simulink model "CruiseControlMode"  (R2022b)
settings: Solver=FixedStepDiscrete  StartTime=0.0  StopTime=10.0  FixedStep=0.01  RelTol=1e-3
undefined symbols (not defined in the file or in its folder): brake_threshold, KeyON, opMode, reqMode, ShiftDrive, tsp_max, tsp_min
libraries: simulink x46
settings Model: RequirementInfo={} %GIDa_d2754c3b_5e37_4166_8f7d_123f4ab94d38  DataDictionary=crs_controllerdic.sldd  EnableAccessToBaseWorkspace=off  Creator=The MathWorks, Inc.  LastModifiedBy=KSREERANG
settings SolverCC: AlgebraicLoopSolver=TrustRegion
settings DataIOCC: SaveOutput=off  SignalLogging=off  DSMLogging=off  SaveTime=off  ReturnWorkspaceOutputs=off
settings OptimizationCC: DefaultParameterBehavior=Inlined  PassReuseOutputArgsAs=Individual arguments  EfficientTunableParamExpr=on
settings DebuggingCC: ParameterTunabilityLossMsg=error  UnconnectedInputMsg=warning  UnconnectedOutputMsg=warning  UnconnectedLineMsg=warning  SFMachineParentedDataDiag=warning  ArithmeticOperatorsInVariantConditions=warning
settings ModelReferenceCC: EnableRefExpFcnMdlSchedulingChecks=on
settings SFSimCC: SimUseLocalCustomCode=off  CustomCodeUndefinedFunction=UseInterfaceOnly
settings RTWCC: Description=Embedded Coder  SystemTargetFile=ert.tlc  GenCodeOnly=on  TemplateMakefile=ert_default_tmf  GenerateReport=on  RTWUseLocalCustomCode=off  IncludeHyperlinkInReport=on  LaunchReport=on  GenerateTraceInfo=on  GenerateTraceReport=on  GenerateTraceReportSl=on  GenerateTraceReportSf=on  GenerateTraceReportEml=on  DLArmComputeVersion=19.05
settings CodeAppCC: ForceParamTrailComments=on  IgnoreCustomStorageClasses=off  OperatorAnnotations=on  SimulinkDataObjDesc=on  SFDataObjDesc=on  MATLABFcnDesc=on  InsertBlockDesc=on  StateflowObjectComments=on  MATLABSourceComments=on  ReqsInCode=on
settings ERTTargetCC: TargetLangStandard=C99 (ISO)  GenerateSampleERTMain=on  InlinedParameterPlacement=NonHierarchical  ERTCustomFileTemplate=example_file_process.tlc

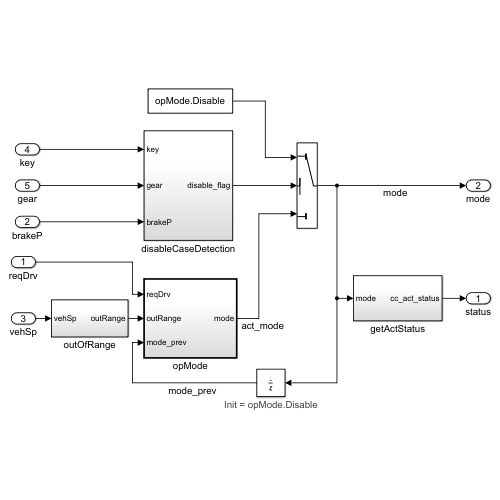
[thumbnail: Simulink's stored preview of the top-level diagram]
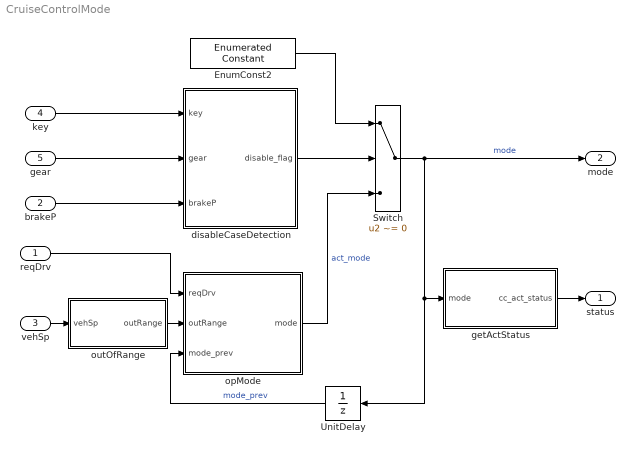
== system CruiseControlMode ==
  reqDrv : Inport  RequirementInfo={} %GIDa_e02c04ea_ec13_49e9_be49_37d1e0b933a9  OutDataTypeStr=Enum: reqMode  PortDimensions=1  SampleTime=[0.01,0]
  brakeP : Inport  RequirementInfo={} %GIDa_3b7b0db5_0c42_456e_bffc_824e0e006553  Port=2  OutDataTypeStr=double  PortDimensions=1  SampleTime=[0.01,0]
  vehSp : Inport  RequirementInfo={} %GIDa_87056838_1774_4720_931e_310af0b5e184  Port=3  OutDataTypeStr=double  PortDimensions=1  SampleTime=[0.01,0]
  key : Inport  RequirementInfo={} %GIDa_da618038_e4b4_4630_9454_d4f85815a96a  Port=4  OutDataTypeStr=uint8  PortDimensions=1  SampleTime=[0.01,0]
  gear : Inport  RequirementInfo={} %GIDa_417b91ae_b290_4c6e_bd19_c183e206983d  Port=5  OutDataTypeStr=uint8  PortDimensions=1  SampleTime=[0.01,0]
  EnumConst2 : simulink/Sources/Enumerated Constant  OutDataTypeStr=Enum: opMode  Value=opMode.Disable  SampleTime=inf
  Switch : Switch  RequirementInfo={} %GIDa_134f0e30_122b_43c5_8efc_d29582d40c21  Criteria=u2 ~= 0  SaturateOnIntegerOverflow=off  InputSameDT=off
  UnitDelay : UnitDelay  RequirementInfo={} %GIDa_6cca9198_01f1_4570_b07c_de3761ab8219  InitialCondition=opMode.Disable  SampleTime=-1  HasFrameUpgradeWarning=on
      settings: AttributesFormatString=Init = %<InitialCondition>
  disableCaseDetection : Subsystem  RequirementInfo={} %GIDa_30cfa19a_c319_430d_857b_86cf10c70b3e
  getActStatus : Subsystem  RequirementInfo={} %GIDa_922b883f_e498_4622_88f6_724ffdd11509
  opMode : Subsystem  RequirementInfo={} %GIDa_e315da79_f503_4e3a_a896_f4bec06d1909  TreatAsAtomicUnit=on
  outOfRange : Subsystem  RequirementInfo={} %GIDa_6a8018be_f3b6_456e_9531_311e94e8f57d
  status : Outport  RequirementInfo={} %GIDa_0f94b556_bb21_4013_9d6a_be506c43a1e9  OutDataTypeStr=boolean  PortDimensions=1  SampleTime=[0.01,0]  VectorParamsAs1DForOutWhenUnconnected=off
  mode : Outport  RequirementInfo={} %GIDa_cedbaee0_5a22_4a89_bb43_144b8d7ba06b  Port=2  OutDataTypeStr=Enum: opMode  PortDimensions=1  SampleTime=[0.01,0]  VectorParamsAs1DForOutWhenUnconnected=off
  wires:
  EnumConst2/1 -> Switch/1
  brakeP/1 -> disableCaseDetection/3(brakeP)
  key/1 -> disableCaseDetection/1(key)
  gear/1 -> disableCaseDetection/2(gear)
  disableCaseDetection/1(disable_flag) -> Switch/2
  reqDrv/1 -> opMode/1(reqDrv)
  UnitDelay/1 -> opMode/3(mode_prev)  "mode_prev"
  getActStatus/1(cc_act_status) -> status/1
  opMode/1(mode) -> Switch/3  "act_mode"
  Switch/1 -> UnitDelay/1, getActStatus/1(mode), mode/1  "mode"
  vehSp/1 -> outOfRange/1(vehSp)
  outOfRange/1(outRange) -> opMode/2(outRange)

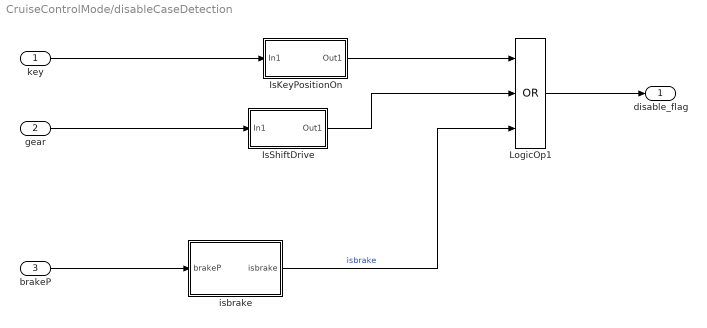
== system CruiseControlMode/disableCaseDetection ==
  key : Inport  RequirementInfo={} %GIDa_c582e8bc_b654_4724_afb0_c4fc2a3f6909
  gear : Inport  RequirementInfo={} %GIDa_4cb0485d_973c_48c3_a789_740fa1fc93bd  Port=2
  brakeP : Inport  RequirementInfo={} %GIDa_84889384_43e7_4e09_aa08_16226f740df6  Port=3
  IsKeyPositionOn : Subsystem  RequirementInfo={} %GIDa_5fa75b47_70b0_4656_b72f_350de8951d87
  IsShiftDrive : Subsystem  RequirementInfo={} %GIDa_d1da0970_5a6e_4cfb_b99c_ed1fdadca6ff
  LogicOp1 : Logic  RequirementInfo={} %GIDa_0e7638fa_faba_4642_af12_693558d1e7f2  Operator=OR  Inputs=3  AllPortsSameDT=off  OutDataTypeStr=boolean
  isbrake : Subsystem  RequirementInfo={} %GIDa_c5463be8_f4ae_4cec_a339_b8202d63dca3
  disable_flag : Outport  RequirementInfo={} %GIDa_06062790_d1b3_4bb4_a6b4_14f289277b04  VectorParamsAs1DForOutWhenUnconnected=off
  wires:
  IsShiftDrive/1(Out1) -> LogicOp1/2
  gear/1 -> IsShiftDrive/1(In1)
  IsKeyPositionOn/1(Out1) -> LogicOp1/1
  key/1 -> IsKeyPositionOn/1(In1)
  isbrake/1(isbrake) -> LogicOp1/3  "isbrake"
  brakeP/1 -> isbrake/1(brakeP)
  LogicOp1/1 -> disable_flag/1

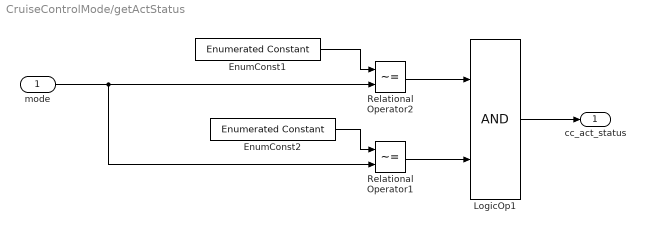
== system CruiseControlMode/getActStatus ==
  mode : Inport  RequirementInfo={} %GIDa_2327d0a8_9f89_4824_af80_f140e8b7cb64
  EnumConst1 : simulink/Sources/Enumerated Constant  RequirementInfo={} %GIDa_f8aa3c76_e1da_47ae_9bc1_37456c4f810e  OutDataTypeStr=Enum: opMode  Value=opMode.Disable  SampleTime=inf
  EnumConst2 : simulink/Sources/Enumerated Constant  RequirementInfo={} %GIDa_73c92ee3_ccad_4e01_ae3b_3441c492584d  OutDataTypeStr=Enum: opMode  Value=opMode.Enable  SampleTime=inf
  LogicOp1 : Logic  RequirementInfo={} %GIDa_d1891a75_3176_4f01_b4a6_061b63f5b5e7  AllPortsSameDT=off  OutDataTypeStr=boolean
  Relational Operator1 : RelationalOperator  RequirementInfo={} %GIDa_0ac04840_0dbf_4a47_a92d_a07906c67fea  Operator=~=  OutDataTypeStr=boolean  InputSameDT=off
  Relational Operator2 : RelationalOperator  RequirementInfo={} %GIDa_da8b8f51_89d3_4582_904d_6d29522943a4  Operator=~=  OutDataTypeStr=boolean  InputSameDT=off
  cc_act_status : Outport  RequirementInfo={} %GIDa_4f6d64e4_ebde_4261_a75c_bc573f921507  VectorParamsAs1DForOutWhenUnconnected=off
  wires:
  LogicOp1/1 -> cc_act_status/1
  EnumConst2/1 -> Relational Operator1/1
  Relational Operator1/1 -> LogicOp1/2
  mode/1 -> Relational Operator2/2, Relational Operator1/2
  EnumConst1/1 -> Relational Operator2/1
  Relational Operator2/1 -> LogicOp1/1

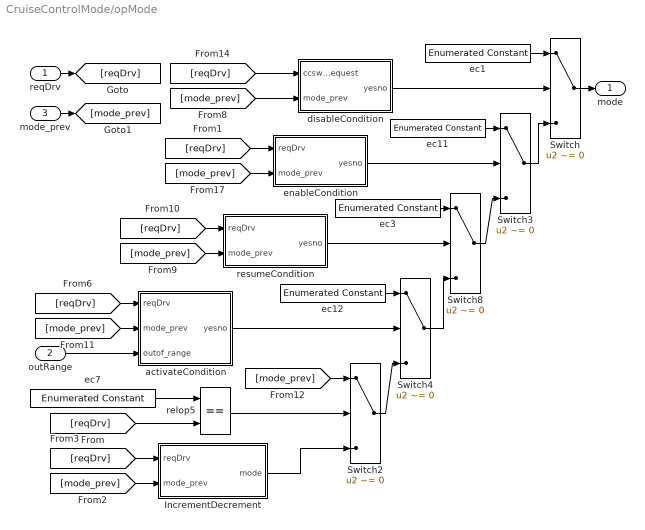
== system CruiseControlMode/opMode ==
  reqDrv : Inport  RequirementInfo={} %GIDa_d6dc1c84_5b93_4ebd_a6cb_51c4e313a83b
  outRange : Inport  RequirementInfo={} %GIDa_8f85a2d2_ead7_4273_a37e_68fc2be8b446  Port=2
  mode_prev : Inport  RequirementInfo={} %GIDa_f8adc632_9c19_43ab_ab94_9239398279c8  Port=3
  IncrementDecrement : Subsystem  RequirementInfo={} %GIDa_cf4f9597_e849_4031_bd26_eb00965c4499
  Switch : Switch  RequirementInfo={} %GIDa_f278f199_6b25_4f5b_af21_e9d29d6a7a0f  Criteria=u2 ~= 0  SaturateOnIntegerOverflow=off  InputSameDT=off
  Switch2 : Switch  RequirementInfo={} %GIDa_e275915e_0819_4e2f_a4fa_10d11a8f267d  Criteria=u2 ~= 0  SaturateOnIntegerOverflow=off  InputSameDT=off
  Switch3 : Switch  RequirementInfo={} %GIDa_e58e5032_d959_406a_99aa_4681a14fd21b  Criteria=u2 ~= 0  SaturateOnIntegerOverflow=off  InputSameDT=off
  Switch4 : Switch  RequirementInfo={} %GIDa_e86cdaa4_f011_4da8_8c69_5ad1193619c6  Criteria=u2 ~= 0  SaturateOnIntegerOverflow=off  InputSameDT=off
  Switch8 : Switch  RequirementInfo={} %GIDa_db82ae89_74d8_429e_a2c1_70767e727218  Criteria=u2 ~= 0  SaturateOnIntegerOverflow=off  InputSameDT=off
  activateCondition : Subsystem  RequirementInfo={} %GIDa_3a1937b1_e63c_4edf_b9e4_c891f61b7724
  disableCondition : Subsystem  RequirementInfo={} %GIDa_f9200ea0_df0d_4770_99ca_2bc3e49d1fe1
  ec1 : simulink/Sources/Enumerated Constant  RequirementInfo={} %GIDa_015a4b04_79f2_421f_ade4_4409e02da5c7  OutDataTypeStr=Enum: opMode  Value=opMode.Disable  SampleTime=inf
  ec11 : simulink/Sources/Enumerated Constant  RequirementInfo={} %GIDa_ec3fa4e4_42ea_4ae3_93ed_8aee2c0a39ed  OutDataTypeStr=Enum: opMode  Value=opMode.Enable  SampleTime=inf
  ec12 : simulink/Sources/Enumerated Constant  RequirementInfo={} %GIDa_fcb4c8b2_4022_407c_87a6_a915c151313b  OutDataTypeStr=Enum: opMode  Value=opMode.Activate  SampleTime=inf
  ec3 : simulink/Sources/Enumerated Constant  RequirementInfo={} %GIDa_eb9bf327_13fe_48a0_b323_af6e76e203bb  OutDataTypeStr=Enum: opMode  Value=opMode.Resume  SampleTime=inf
  ec7 : simulink/Sources/Enumerated Constant  RequirementInfo={} %GIDa_58ab4a78_7813_419b_8fc1_7974d688ddc1  OutDataTypeStr=Enum: reqMode  Value=reqMode.NoRequest  SampleTime=inf
  enableCondition : Subsystem  RequirementInfo={} %GIDa_2fd9b1f7_d568_4f68_81be_1b30c1f938c3
  relop5 : RelationalOperator  RequirementInfo={} %GIDa_b4c8cdd0_d61d_4e26_84e3_ca073b38d041  Operator===  OutDataTypeStr=boolean  InputSameDT=off
  resumeCondition : Subsystem  RequirementInfo={} %GIDa_a20f1591_47de_4d21_9f12_3ebad1f0684e
  mode : Outport  RequirementInfo={} %GIDa_b396453e_df28_4809_a65d_b57fb24c4239  VectorParamsAs1DForOutWhenUnconnected=off
  wires:
  IncrementDecrement/1(mode) -> Switch2/3
  [mode_prev] -> IncrementDecrement/2(mode_prev)
  [reqDrv] -> IncrementDecrement/1(reqDrv)
  [mode_prev] -> enableCondition/2(mode_prev)
  outRange/1 -> activateCondition/3(outof_range)
  [reqDrv] -> disableCondition/1(ccsw_request)
  ec3/1 -> Switch8/1
  [reqDrv] -> resumeCondition/1(reqDrv)
  [mode_prev] -> resumeCondition/2(mode_prev)
  resumeCondition/1(yesno) -> Switch8/2
  Switch4/1 -> Switch8/3
  Switch8/1 -> Switch3/3
  Switch2/1 -> Switch4/3
  relop5/1 -> Switch2/2
  reqDrv/1 -> [reqDrv]
  [mode_prev] -> disableCondition/2(mode_prev)
  [mode_prev] -> activateCondition/2(mode_prev)
  [reqDrv] -> activateCondition/1(reqDrv)
  activateCondition/1(yesno) -> Switch4/2
  Switch3/1 -> Switch/3
  disableCondition/1(yesno) -> Switch/2
  enableCondition/1(yesno) -> Switch3/2
  mode_prev/1 -> [mode_prev]
  [reqDrv] -> enableCondition/1(reqDrv)
  [mode_prev] -> Switch2/1
  [reqDrv] -> relop5/2
  ec12/1 -> Switch4/1
  ec11/1 -> Switch3/1
  ec7/1 -> relop5/1
  ec1/1 -> Switch/1
  Switch/1 -> mode/1

== system CruiseControlMode/outOfRange ==
  vehSp : Inport  RequirementInfo={} %GIDa_10d93d9c_c07d_4af0_b3dc_570db8225146
  Compare To Constant : simulink/Logic and Bit Operations/Compare To Constant  RequirementInfo={} %GIDa_16aaa0c8_a2f0_4c5a_ae90_6ea610de385c  relop=<  const=tsp_min  OutDataTypeStr=boolean
  Compare To Constant1 : simulink/Logic and Bit Operations/Compare To Constant  RequirementInfo={} %GIDa_bc322242_d9a7_47fb_8ec0_04de03b57b5d  relop=>  const=tsp_max  OutDataTypeStr=boolean
  LogicOp : Logic  RequirementInfo={} %GIDa_9879b928_48e1_4dc2_86e7_6ea8d95ea2bf  Operator=OR  AllPortsSameDT=off  OutDataTypeStr=boolean
  outRange : Outport  RequirementInfo={} %GIDa_05b9ac4e_46b0_439f_8ec8_ced6dca6f32b  VectorParamsAs1DForOutWhenUnconnected=off
  wires:
  vehSp/1 -> Compare To Constant1/1, Compare To Constant/1
  Compare To Constant/1 -> LogicOp/1
  Compare To Constant1/1 -> LogicOp/2
  LogicOp/1 -> outRange/1

== system CruiseControlMode/disableCaseDetection/IsKeyPositionOn ==
  In1 : Inport  RequirementInfo={} %GIDa_fbade00e_be87_4b7c_96f1_342a649bf32e
  Constant : Constant  RequirementInfo={} %GIDa_c80b2359_4f79_4558_8249_60fbc73dc217  Value=KeyON
  Relational Operator2 : RelationalOperator  RequirementInfo={} %GIDa_1085da51_22c4_4519_8a44_d44051c23fa5  Operator=~=  OutDataTypeStr=boolean  InputSameDT=off
  Out1 : Outport  RequirementInfo={} %GIDa_53421d23_320b_4638_b85c_7031813788c3  VectorParamsAs1DForOutWhenUnconnected=off
  wires:
  Constant/1 -> Relational Operator2/2
  In1/1 -> Relational Operator2/1
  Relational Operator2/1 -> Out1/1

== system CruiseControlMode/disableCaseDetection/IsShiftDrive ==
  In1 : Inport  RequirementInfo={} %GIDa_e638b041_459c_4a49_806d_2e8e8e3b1d25
  Constant1 : Constant  RequirementInfo={} %GIDa_728aeb5c_840b_4b38_9d35_2bb658e3a343  Value=ShiftDrive
  Relational Operator3 : RelationalOperator  RequirementInfo={} %GIDa_8fff1215_8b51_4cbc_a454_5baa57c7c947  Operator=~=  OutDataTypeStr=boolean  InputSameDT=off
  Out1 : Outport  RequirementInfo={} %GIDa_bd684801_c897_47ac_8c54_81cdc672ae87  VectorParamsAs1DForOutWhenUnconnected=off
  wires:
  Constant1/1 -> Relational Operator3/2
  In1/1 -> Relational Operator3/1
  Relational Operator3/1 -> Out1/1

== system CruiseControlMode/disableCaseDetection/isbrake ==
  brakeP : Inport  RequirementInfo={} %GIDa_39c608f7_59ae_4c31_a873_5a7787b80baa
  Compare To Constant : simulink/Logic and Bit Operations/Compare To Constant  RequirementInfo={} %GIDa_189ea09c_3f5c_40b7_82bc_4cba1ee5f74b  relop=>  const=brake_threshold  OutDataTypeStr=boolean
  isbrake : Outport  RequirementInfo={} %GIDa_5b8aaf44_fb4f_460a_80ba_c6eab77b7a44  VectorParamsAs1DForOutWhenUnconnected=off
  wires:
  Compare To Constant/1 -> isbrake/1
  brakeP/1 -> Compare To Constant/1

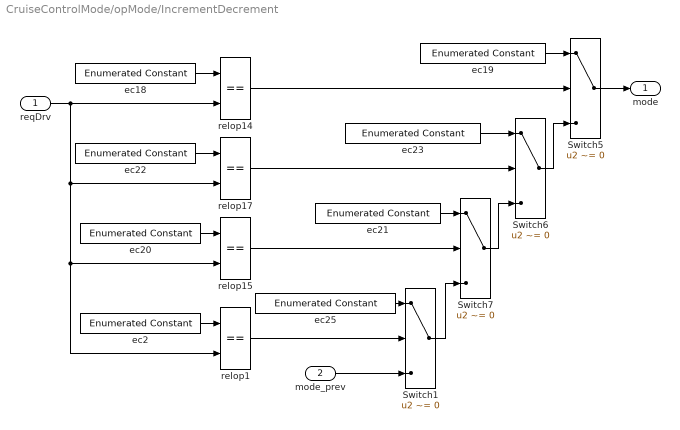
== system CruiseControlMode/opMode/IncrementDecrement ==
  reqDrv : Inport  RequirementInfo={} %GIDa_e2bc38eb_5ae3_43b9_a114_d74f24c6e37b
  mode_prev : Inport  RequirementInfo={} %GIDa_5373f4eb_c723_4fec_a619_dc0302e64efa  Port=2
  Switch1 : Switch  RequirementInfo={} %GIDa_3da03518_a025_4b01_9142_099afa888f0e  Criteria=u2 ~= 0  SaturateOnIntegerOverflow=off  InputSameDT=off
  Switch5 : Switch  RequirementInfo={} %GIDa_ad15e83e_a1a5_494f_97a5_7e76ad4b6e6a  Criteria=u2 ~= 0  SaturateOnIntegerOverflow=off  InputSameDT=off
  Switch6 : Switch  RequirementInfo={} %GIDa_d7f0e410_c4f9_4851_913e_6272620f0d58  Criteria=u2 ~= 0  SaturateOnIntegerOverflow=off  InputSameDT=off
  Switch7 : Switch  RequirementInfo={} %GIDa_76c38470_6d2c_4821_909c_522b3827856b  Criteria=u2 ~= 0  SaturateOnIntegerOverflow=off  InputSameDT=off
  ec18 : simulink/Sources/Enumerated Constant  RequirementInfo={} %GIDa_1f657265_3a4b_4f99_8045_e03baf4bd613  OutDataTypeStr=Enum: reqMode  Value=reqMode.Inc_Short  SampleTime=inf
  ec19 : simulink/Sources/Enumerated Constant  RequirementInfo={} %GIDa_da36edf3_ca28_44dd_9c44_3816caf78137  OutDataTypeStr=Enum: opMode  Value=opMode.Increment  SampleTime=inf
  ec2 : simulink/Sources/Enumerated Constant  RequirementInfo={} %GIDa_9273ddb4_1d3b_443f_98f7_4d2b24f19bc0  OutDataTypeStr=Enum: reqMode  Value=reqMode.Dec_Long  SampleTime=inf
  ec20 : simulink/Sources/Enumerated Constant  RequirementInfo={} %GIDa_795dac68_6a3a_4e07_affa_8c2c129b871d  OutDataTypeStr=Enum: reqMode  Value=reqMode.Dec_Short  SampleTime=inf
  ec21 : simulink/Sources/Enumerated Constant  RequirementInfo={} %GIDa_b5dc6f1e_17b1_4531_8089_3a1730281df9  OutDataTypeStr=Enum: opMode  Value=opMode.Decrement  SampleTime=inf
  ec22 : simulink/Sources/Enumerated Constant  RequirementInfo={} %GIDa_6acb6ee2_ef5b_4345_84a3_9181b47d18e8  OutDataTypeStr=Enum: reqMode  Value=reqMode.Inc_Long  SampleTime=inf
  ec23 : simulink/Sources/Enumerated Constant  RequirementInfo={} %GIDa_18759121_a88a_4695_aba9_877ce84448f2  OutDataTypeStr=Enum: opMode  Value=opMode.IncrementHold  SampleTime=inf
  ec25 : simulink/Sources/Enumerated Constant  RequirementInfo={} %GIDa_0fe9807b_c2cf_4c75_9774_a51ab4388cde  OutDataTypeStr=Enum: opMode  Value=opMode.DecrementHold  SampleTime=inf
  relop1 : RelationalOperator  RequirementInfo={} %GIDa_e875ba4b_a404_460a_9e1b_b0d1157735d3  Operator===  OutDataTypeStr=boolean  InputSameDT=off
  relop14 : RelationalOperator  RequirementInfo={} %GIDa_a828a7b6_80d5_4932_a549_e889a70ae76f  Operator===  OutDataTypeStr=boolean  InputSameDT=off
  relop15 : RelationalOperator  RequirementInfo={} %GIDa_a3f1fb2c_be05_49f4_b0d8_78a17c2da26b  Operator===  OutDataTypeStr=boolean  InputSameDT=off
  relop17 : RelationalOperator  RequirementInfo={} %GIDa_ea05844d_1ae3_4b99_85d9_44a8123c96a9  Operator===  OutDataTypeStr=boolean  InputSameDT=off
  mode : Outport  RequirementInfo={} %GIDa_5d5012d3_58ac_4298_b4d7_8a2f3101ae51  VectorParamsAs1DForOutWhenUnconnected=off
  wires:
  reqDrv/1 -> relop14/2, relop17/2, relop15/2, relop1/2
  Switch5/1 -> mode/1
  relop14/1 -> Switch5/2
  ec18/1 -> relop14/1
  mode_prev/1 -> Switch1/3
  relop1/1 -> Switch1/2
  ec2/1 -> relop1/1
  Switch1/1 -> Switch7/3
  ec25/1 -> Switch1/1
  Switch7/1 -> Switch6/3
  ec21/1 -> Switch7/1
  relop15/1 -> Switch7/2
  ec20/1 -> relop15/1
  Switch6/1 -> Switch5/3
  ec23/1 -> Switch6/1
  relop17/1 -> Switch6/2
  ec22/1 -> relop17/1
  ec19/1 -> Switch5/1

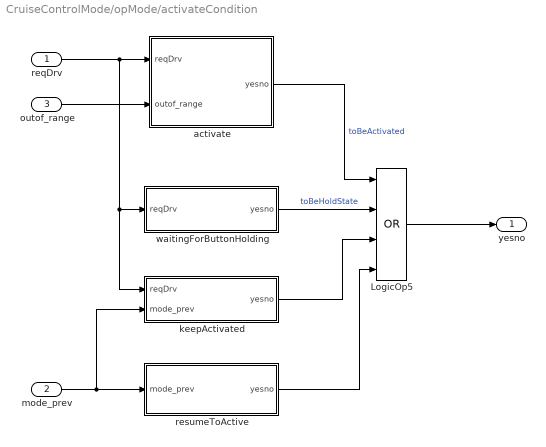
== system CruiseControlMode/opMode/activateCondition ==
  reqDrv : Inport  RequirementInfo={} %GIDa_15fdfca6_8f0c_489b_a680_659e7f1acd40
  mode_prev : Inport  RequirementInfo={} %GIDa_375ed21a_680e_4188_b39c_14c0b0419ce3  Port=2
  outof_range : Inport  RequirementInfo={} %GIDa_ccbb498a_39dc_42aa_9748_b1fab1679509  Port=3
  LogicOp5 : Logic  RequirementInfo={} %GIDa_1f1f3340_53a8_4cf3_aba1_6d6d2f2a7d3a  Operator=OR  Inputs=4  AllPortsSameDT=off  OutDataTypeStr=boolean
  activate : Subsystem  RequirementInfo={} %GIDa_ae753962_f36b_4896_8190_9ff64202b598
  keepActivated : Subsystem  RequirementInfo={} %GIDa_31cdea4a_4fb3_477d_beaa_8c8bfca90bc0
  resumeToActive : Subsystem  RequirementInfo={} %GIDa_52ef6869_8b8a_4a88_97e9_527087414cdd
  waitingForButtonHolding : Subsystem  RequirementInfo={} %GIDa_d152685c_bd82_4fc3_8902_76004ba249e5
  yesno : Outport  RequirementInfo={} %GIDa_a451725f_a3c6_4912_923c_f002f163403e  VectorParamsAs1DForOutWhenUnconnected=off
  wires:
  mode_prev/1 -> resumeToActive/1(mode_prev), keepActivated/2(mode_prev)
  resumeToActive/1(yesno) -> LogicOp5/4
  activate/1(yesno) -> LogicOp5/1  "toBeActivated"
  waitingForButtonHolding/1(yesno) -> LogicOp5/2  "toBeHoldState"
  keepActivated/1(yesno) -> LogicOp5/3
  outof_range/1 -> activate/2(outof_range)
  LogicOp5/1 -> yesno/1
  reqDrv/1 -> activate/1(reqDrv), waitingForButtonHolding/1(reqDrv), keepActivated/1(reqDrv)

== system CruiseControlMode/opMode/disableCondition ==
  ccsw_request : Inport  RequirementInfo={} %GIDa_b101258d_165d_4d04_82f5_55b581071af0
  mode_prev : Inport  RequirementInfo={} %GIDa_6cc3844b_31a9_4b0f_9f1e_2073909f59a1  Port=2
  LogicOp7 : Logic  RequirementInfo={} %GIDa_ce563152_e3e7_4710_94ca_17a1ff19942b  Operator=OR  AllPortsSameDT=off  OutDataTypeStr=boolean
  buttonsShouldBeCalledWhenActivated : Subsystem  RequirementInfo={} %GIDa_454b6547_c400_48f4_a548_bf377e739686
  turnOffCruise : Subsystem  RequirementInfo={} %GIDa_28458284_b25f_4ba6_ba6a_dfac332ba428
  yesno : Outport  RequirementInfo={} %GIDa_58737c6d_d13a_4674_9c00_2cb4f5887bd5  VectorParamsAs1DForOutWhenUnconnected=off
  wires:
  buttonsShouldBeCalledWhenActivated/1(yesno) -> LogicOp7/2
  turnOffCruise/1(yesno) -> LogicOp7/1
  mode_prev/1 -> turnOffCruise/2(mode_prev), buttonsShouldBeCalledWhenActivated/2(mode_prev)
  LogicOp7/1 -> yesno/1
  ccsw_request/1 -> turnOffCruise/1(ccsw_request), buttonsShouldBeCalledWhenActivated/1(ccsw_request)

== system CruiseControlMode/opMode/enableCondition ==
  reqDrv : Inport  RequirementInfo={} %GIDa_2ea5ef3a_8075_494a_b65a_a486881d86e0
  mode_prev : Inport  RequirementInfo={} %GIDa_64fc3c2f_a7ba_46f0_a281_7c33f1d21fa0  Port=2
  LogicOp4 : Logic  RequirementInfo={} %GIDa_46bf2960_6ddb_4fdf_b265_cd063c6e6a6c  Operator=OR  AllPortsSameDT=off  OutDataTypeStr=boolean
  cancelActivation : Subsystem  RequirementInfo={} %GIDa_159434b1_1c3d_4a15_9aa0_8458f8422ce8
  pressSetSw : Subsystem  RequirementInfo={} %GIDa_fbd60129_0c32_4cf4_9077_6b4ce66fdda5
  yesno : Outport  RequirementInfo={} %GIDa_fc0b228d_7017_44e3_82c8_d38ebd747cda  VectorParamsAs1DForOutWhenUnconnected=off
  wires:
  pressSetSw/1(yesno) -> LogicOp4/1
  mode_prev/1 -> cancelActivation/2(mode_prev)
  cancelActivation/1(yesno) -> LogicOp4/2
  reqDrv/1 -> pressSetSw/1(reqDrv), cancelActivation/1(reqDrv)
  LogicOp4/1 -> yesno/1

== system CruiseControlMode/opMode/resumeCondition ==
  reqDrv : Inport  RequirementInfo={} %GIDa_dd8f4abc_ebf9_4119_9cf7_de93c1f76bab
  mode_prev : Inport  RequirementInfo={} %GIDa_cc6596f2_c8cf_4065_a552_ab3a57f275ec  Port=2
  LogicOp6 : Logic  RequirementInfo={} %GIDa_ab105c5e_d731_4be9_8ecd_c885bab9cf08  AllPortsSameDT=off  OutDataTypeStr=boolean
  enableToResume : Subsystem  RequirementInfo={} %GIDa_7179038e_fcf9_48eb_955f_73dabda87ba3
  hasCanceled : Subsystem  RequirementInfo={} %GIDa_3a04595b_c0bd_4643_b117_9ef470d38a2f
  yesno : Outport  RequirementInfo={} %GIDa_76586af4_82d8_4d43_a25e_8aa98b22a9c3  VectorParamsAs1DForOutWhenUnconnected=off
  wires:
  reqDrv/1 -> enableToResume/1(reqDrv)
  enableToResume/1(yesno) -> LogicOp6/1
  hasCanceled/1(yesno) -> LogicOp6/2
  mode_prev/1 -> hasCanceled/1(mode_prev), enableToResume/2(mode_prev)
  LogicOp6/1 -> yesno/1

== system CruiseControlMode/opMode/activateCondition/activate ==
  reqDrv : Inport  RequirementInfo={} %GIDa_92021680_f573_4b71_beef_de1d77884918
  outof_range : Inport  RequirementInfo={} %GIDa_b33e8474_cae9_4251_81f7_45bab2d7408c  Port=2
  LogicOp3 : Logic  RequirementInfo={} %GIDa_f478c711_7841_4b54_ac61_bcc2dd24a464  AllPortsSameDT=off  OutDataTypeStr=boolean
  LogicOp5 : Logic  RequirementInfo={} %GIDa_fc73e6c1_3fec_4021_b1f7_5215957fe166  Operator=NOT  AllPortsSameDT=off  OutDataTypeStr=boolean
  ec15 : simulink/Sources/Enumerated Constant  RequirementInfo={} %GIDa_0e5a3865_a76c_42df_bf63_01cd05cb4a71  OutDataTypeStr=Enum: reqMode  Value=reqMode.Set  SampleTime=inf
  relop11 : RelationalOperator  RequirementInfo={} %GIDa_5d308316_c777_48ea_a859_6533c44b1cab  Operator===  OutDataTypeStr=boolean  InputSameDT=off
  yesno : Outport  RequirementInfo={} %GIDa_c8e3f60d_f268_421b_a0f2_3fb47ff7ff7e  VectorParamsAs1DForOutWhenUnconnected=off
  wires:
  LogicOp5/1 -> LogicOp3/2
  outof_range/1 -> LogicOp5/1
  relop11/1 -> LogicOp3/1
  LogicOp3/1 -> yesno/1
  reqDrv/1 -> relop11/2
  ec15/1 -> relop11/1

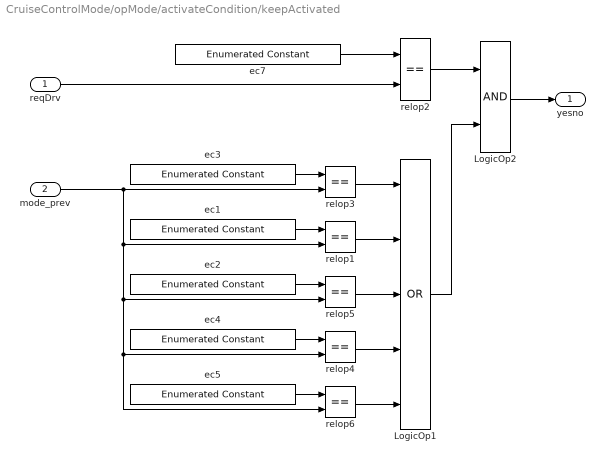
== system CruiseControlMode/opMode/activateCondition/keepActivated ==
  reqDrv : Inport  RequirementInfo={} %GIDa_23e2775e_9aa6_450b_98b5_97c4514ff2d1
  mode_prev : Inport  RequirementInfo={} %GIDa_412ed595_3f68_4805_9d7b_e9a96f949d90  Port=2
  LogicOp1 : Logic  RequirementInfo={} %GIDa_b07aa5d9_ecaf_49a2_997b_df751528869f  Operator=OR  Inputs=5  AllPortsSameDT=off  OutDataTypeStr=boolean
  LogicOp2 : Logic  RequirementInfo={} %GIDa_b368a1b2_d1c4_4d1c_af15_c0c18290571a  AllPortsSameDT=off  OutDataTypeStr=boolean
  ec1 : simulink/Sources/Enumerated Constant  RequirementInfo={} %GIDa_4d3a5127_e183_4e47_b7de_98a6ba0455ca  OutDataTypeStr=Enum: opMode  Value=opMode.Increment  SampleTime=inf
  ec2 : simulink/Sources/Enumerated Constant  RequirementInfo={} %GIDa_eece2236_d9d8_4e92_ae65_d6331a28a99c  OutDataTypeStr=Enum: opMode  Value=opMode.IncrementHold  SampleTime=inf
  ec3 : simulink/Sources/Enumerated Constant  RequirementInfo={} %GIDa_c9b1ff48_3104_429a_a9f2_8e2b0046d60a  OutDataTypeStr=Enum: opMode  Value=opMode.Activate  SampleTime=inf
  ec4 : simulink/Sources/Enumerated Constant  RequirementInfo={} %GIDa_1333e43c_0fd1_46f8_b4ee_95aa609fb605  OutDataTypeStr=Enum: opMode  Value=opMode.Decrement  SampleTime=inf
  ec5 : simulink/Sources/Enumerated Constant  RequirementInfo={} %GIDa_c0dc8051_d9cd_4b58_8add_0d9e2cb2294b  OutDataTypeStr=Enum: opMode  Value=opMode.DecrementHold  SampleTime=inf
  ec7 : simulink/Sources/Enumerated Constant  RequirementInfo={} %GIDa_5b86c125_f995_4152_89db_377e46efbcc7  OutDataTypeStr=Enum: reqMode  Value=reqMode.NoRequest  SampleTime=inf
  relop1 : RelationalOperator  RequirementInfo={} %GIDa_14a62092_02f0_4f36_b093_1db4d941d800  Operator===  OutDataTypeStr=boolean  InputSameDT=off
  relop2 : RelationalOperator  RequirementInfo={} %GIDa_44c2a5b1_1200_49e6_bfd1_5656d91a32b2  Operator===  OutDataTypeStr=boolean  InputSameDT=off
  relop3 : RelationalOperator  RequirementInfo={} %GIDa_f41a4325_378c_4a3d_a901_a943ad83ed09  Operator===  OutDataTypeStr=boolean  InputSameDT=off
  relop4 : RelationalOperator  RequirementInfo={} %GIDa_19d07942_2349_444d_9916_9212e6cea081  Operator===  OutDataTypeStr=boolean  InputSameDT=off
  relop5 : RelationalOperator  RequirementInfo={} %GIDa_e89d4640_46d9_4537_9137_3b57f2522c07  Operator===  OutDataTypeStr=boolean  InputSameDT=off
  relop6 : RelationalOperator  RequirementInfo={} %GIDa_354d344c_94f0_4a4e_b5dd_d4aef05ae917  Operator===  OutDataTypeStr=boolean  InputSameDT=off
  yesno : Outport  RequirementInfo={} %GIDa_3597e7f8_1747_4110_9525_1c491fd67914  VectorParamsAs1DForOutWhenUnconnected=off
  wires:
  LogicOp2/1 -> yesno/1
  reqDrv/1 -> relop2/2
  relop3/1 -> LogicOp1/1
  relop1/1 -> LogicOp1/2
  ec3/1 -> relop3/1
  ec1/1 -> relop1/1
  ec7/1 -> relop2/1
  ec2/1 -> relop5/1
  ec4/1 -> relop4/1
  relop5/1 -> LogicOp1/3
  relop4/1 -> LogicOp1/4
  mode_prev/1 -> relop6/2, relop4/2, relop5/2, relop1/2, relop3/2
  ec5/1 -> relop6/1
  relop6/1 -> LogicOp1/5
  relop2/1 -> LogicOp2/1
  LogicOp1/1 -> LogicOp2/2

== system CruiseControlMode/opMode/activateCondition/resumeToActive ==
  mode_prev : Inport  RequirementInfo={} %GIDa_a1652ed0_ddc2_4599_8fbc_a3925127ba43
  ec3 : simulink/Sources/Enumerated Constant  RequirementInfo={} %GIDa_9100d5f6_4fc5_4875_b858_559b246f23bd  OutDataTypeStr=Enum: opMode  Value=opMode.Resume  SampleTime=inf
  relop2 : RelationalOperator  RequirementInfo={} %GIDa_02ac224a_52db_4e84_885b_4abbec7a7e32  Operator===  OutDataTypeStr=boolean  InputSameDT=off
  yesno : Outport  RequirementInfo={} %GIDa_1f927a13_06ea_4f21_8310_1ececcb0c1c8  VectorParamsAs1DForOutWhenUnconnected=off
  wires:
  relop2/1 -> yesno/1
  ec3/1 -> relop2/1
  mode_prev/1 -> relop2/2

== system CruiseControlMode/opMode/activateCondition/waitingForButtonHolding ==
  reqDrv : Inport  RequirementInfo={} %GIDa_2e2c5b38_9d2a_4e48_9153_04cd6b29a97f
  LogicOp6 : Logic  RequirementInfo={} %GIDa_7712f46c_eba9_4803_933f_c47421edc2b0  Operator=OR  AllPortsSameDT=off  OutDataTypeStr=boolean
  ec10 : Subsystem  RequirementInfo={} %GIDa_165b607b_6770_4492_8ec2_c9d6900211d8  DialogController=Simulink.DDGSource  mask(Enumerated Constant){OutDataTypeStr=Enum: reqMode, Value=reqMode.Dec_Middle, SampleTime=inf}
      mask prompts: OutDataTypeStr "Simulink:blkprm_prompts:OutputDataType"; Value "Simulink:blkprm_prompts:ConstConstValue"; SampleTime "Simulink:blkprm_prompts:AllSrcBlksSampleTime"
      mask init:
      | % NOTE:
      | % Value parameter is not evaluated to avoid caching an instance
      | % of the enumeration class by the mask infrastructure.
      | 
      | % Get expression for OutDataTypeStr before evaluation
      | OutDataTypeStr = get_param(gcbh, 'OutDataTypeStr');
      | 
      | % Check data type & value
      | enumconst_cb('MaskInit', OutDataTypeStr, slResolve(Value, gcb));
      | 
      | % Set mask parameter values directly on underlying block
      | % and clear mask workspace variables to prevent underlying
      | % blocks from resolving to unevaluated mask variables.
      | set_param([gcb, '/Constant'], ...
      |     'OutDataTypeStr', OutDataTypeStr, ...
      |     'SampleTime',     SampleTime, ...
      |     'Value',          Value);
      | clear OutDataTypeStr SampleTime Value;
      mask Display:
      | % Get string to use for display purposes
      | enumConstDispStr = get_param(gcbh, 'Value');
      | if isempty(enumConstDispStr)
      | 
      | 				    end
      | disp(enumConstDispStr)
  ec8 : Subsystem  RequirementInfo={} %GIDa_ee8e63bd_89af_41d0_a2d2_d1ec890d9a81  DialogController=Simulink.DDGSource  mask(Enumerated Constant){OutDataTypeStr=Enum: reqMode, Value=reqMode.Inc_Middle, SampleTime=inf}
      mask prompts: OutDataTypeStr "Simulink:blkprm_prompts:OutputDataType"; Value "Simulink:blkprm_prompts:ConstConstValue"; SampleTime "Simulink:blkprm_prompts:AllSrcBlksSampleTime"
      mask init: same as CruiseControlMode/opMode/activateCondition/waitingForButtonHolding/ec10
      mask Display:
      | % Get string to use for display purposes
      | enumConstDispStr = get_param(gcbh, 'Value');
      | if isempty(enumConstDispStr)
      | 
      | 				    end
      | disp(enumConstDispStr)
  relop10 : RelationalOperator  RequirementInfo={} %GIDa_2c0f799b_2d96_4ee6_acaf_e87a48ddd779  Operator===  OutDataTypeStr=boolean  InputSameDT=off
  relop11 : RelationalOperator  RequirementInfo={} %GIDa_b710b49b_e2dc_4f5a_8c3d_b837515cbc65  Operator===  OutDataTypeStr=boolean  InputSameDT=off
  yesno : Outport  RequirementInfo={} %GIDa_46080d95_bce3_4f08_a6d5_30b811439bf8  VectorParamsAs1DForOutWhenUnconnected=off
  wires:
  LogicOp6/1 -> yesno/1
  reqDrv/1 -> relop11/2, relop10/2
  relop11/1 -> LogicOp6/2
  ec10/1(Out) -> relop11/1
  relop10/1 -> LogicOp6/1
  ec8/1(Out) -> relop10/1

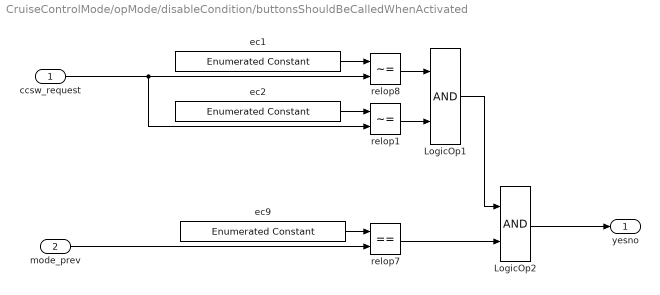
== system CruiseControlMode/opMode/disableCondition/buttonsShouldBeCalledWhenActivated ==
  ccsw_request : Inport  RequirementInfo={} %GIDa_c8726348_d439_477c_a3de_4589f5ea950b
  mode_prev : Inport  RequirementInfo={} %GIDa_01dad347_2b42_436d_91ed_65b2a9a7c83d  Port=2
  LogicOp1 : Logic  RequirementInfo={} %GIDa_2b6aca9c_9b0c_4830_ae4b_b65c34e547b8  AllPortsSameDT=off  OutDataTypeStr=boolean
  LogicOp2 : Logic  RequirementInfo={} %GIDa_f1a0c9e2_f9ea_469a_8261_5f934f0343d1  AllPortsSameDT=off  OutDataTypeStr=boolean
  ec1 : simulink/Sources/Enumerated Constant  RequirementInfo={} %GIDa_9735398e_5e93_4de6_9292_456230e0f373  OutDataTypeStr=Enum: reqMode  Value=reqMode.Cruise  SampleTime=inf
  ec2 : simulink/Sources/Enumerated Constant  RequirementInfo={} %GIDa_541ef6ad_dbc1_4a81_a041_9ba959b25956  OutDataTypeStr=Enum: reqMode  Value=reqMode.Set  SampleTime=inf
  ec9 : simulink/Sources/Enumerated Constant  RequirementInfo={} %GIDa_cca55121_bfba_4d94_989a_9a9e5e71b564  OutDataTypeStr=Enum: opMode  Value=opMode.Disable  SampleTime=inf
  relop1 : RelationalOperator  RequirementInfo={} %GIDa_e22fe7ca_1165_4dce_b8c4_83e765cf7902  Operator=~=  OutDataTypeStr=boolean  InputSameDT=off
  relop7 : RelationalOperator  RequirementInfo={} %GIDa_8fa9e7c9_542b_42a7_8843_75634a1650b6  Operator===  OutDataTypeStr=boolean  InputSameDT=off
  relop8 : RelationalOperator  RequirementInfo={} %GIDa_95bd2af3_7b35_41c0_aa82_fb25cf55b7b6  Operator=~=  OutDataTypeStr=boolean  InputSameDT=off
  yesno : Outport  RequirementInfo={} %GIDa_7d99a7b0_b7f4_4e38_b9c0_9c812d3091d2  VectorParamsAs1DForOutWhenUnconnected=off
  wires:
  ec2/1 -> relop1/1
  relop1/1 -> LogicOp1/2
  ccsw_request/1 -> relop8/2, relop1/2
  mode_prev/1 -> relop7/2
  LogicOp2/1 -> yesno/1
  relop7/1 -> LogicOp2/2
  LogicOp1/1 -> LogicOp2/1
  relop8/1 -> LogicOp1/1
  ec1/1 -> relop8/1
  ec9/1 -> relop7/1

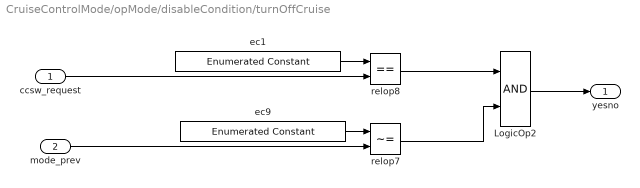
== system CruiseControlMode/opMode/disableCondition/turnOffCruise ==
  ccsw_request : Inport  RequirementInfo={} %GIDa_9c6772b8_5717_435a_a616_0d1ec2bed07a
  mode_prev : Inport  RequirementInfo={} %GIDa_e0664e04_a6c5_4735_af05_ba15f860746e  Port=2
  LogicOp2 : Logic  RequirementInfo={} %GIDa_8143652d_0c06_41c5_b008_bb7ce3d15b1d  AllPortsSameDT=off  OutDataTypeStr=boolean
  ec1 : simulink/Sources/Enumerated Constant  RequirementInfo={} %GIDa_3d51e15b_c494_47b1_8c05_348c7326d085  OutDataTypeStr=Enum: reqMode  Value=reqMode.Cruise  SampleTime=inf
  ec9 : simulink/Sources/Enumerated Constant  RequirementInfo={} %GIDa_6e692d22_f902_4f5f_a37c_3e09a39d9699  OutDataTypeStr=Enum: opMode  Value=opMode.Disable  SampleTime=inf
  relop7 : RelationalOperator  RequirementInfo={} %GIDa_218628e3_e34a_4bf7_b5dd_e9ed0d0c419b  Operator=~=  OutDataTypeStr=boolean  InputSameDT=off
  relop8 : RelationalOperator  RequirementInfo={} %GIDa_731b3793_b8ca_4419_a3b8_294c3bfbf88a  Operator===  OutDataTypeStr=boolean  InputSameDT=off
  yesno : Outport  RequirementInfo={} %GIDa_f8658b70_312f_4b7f_a6e6_7ecc582db363  VectorParamsAs1DForOutWhenUnconnected=off
  wires:
  ec9/1 -> relop7/1
  ec1/1 -> relop8/1
  relop8/1 -> LogicOp2/1
  relop7/1 -> LogicOp2/2
  LogicOp2/1 -> yesno/1
  mode_prev/1 -> relop7/2
  ccsw_request/1 -> relop8/2

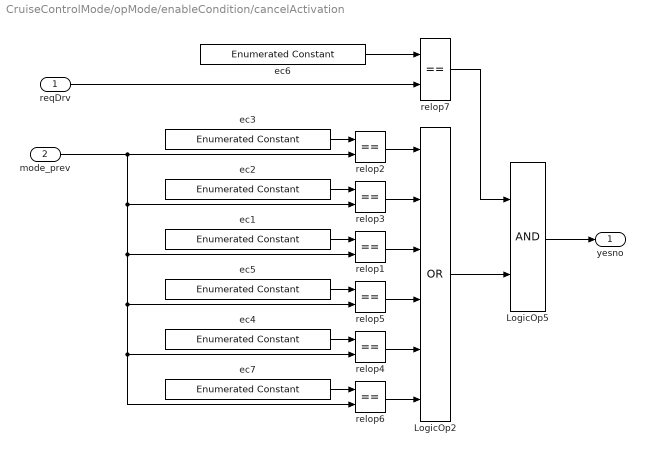
== system CruiseControlMode/opMode/enableCondition/cancelActivation ==
  reqDrv : Inport  RequirementInfo={} %GIDa_294083c2_a080_44d5_b6b3_8751aff424f0
  mode_prev : Inport  RequirementInfo={} %GIDa_9081797a_42d6_4929_97ff_6d66fa4a2386  Port=2
  LogicOp2 : Logic  RequirementInfo={} %GIDa_0a4e3bb1_9057_418e_955e_7bfe6f2d4cf0  Operator=OR  Inputs=6  AllPortsSameDT=off  OutDataTypeStr=boolean
  LogicOp5 : Logic  RequirementInfo={} %GIDa_ef53562d_bbb5_479b_95dd_38c475bd14c7  AllPortsSameDT=off  OutDataTypeStr=boolean
  ec1 : simulink/Sources/Enumerated Constant  RequirementInfo={} %GIDa_cfaf3128_0cc8_4ddf_912c_79abd3664fe6  OutDataTypeStr=Enum: opMode  Value=opMode.IncrementHold  SampleTime=inf
  ec2 : simulink/Sources/Enumerated Constant  RequirementInfo={} %GIDa_5c14bc91_0c92_407f_98e7_edd11f0844cc  OutDataTypeStr=Enum: opMode  Value=opMode.Increment  SampleTime=inf
  ec3 : simulink/Sources/Enumerated Constant  RequirementInfo={} %GIDa_18109c51_61db_4224_adec_b34d8bf6e618  OutDataTypeStr=Enum: opMode  Value=opMode.Activate  SampleTime=inf
  ec4 : simulink/Sources/Enumerated Constant  RequirementInfo={} %GIDa_fda8afc3_260e_4987_87d7_f3266061fd3c  OutDataTypeStr=Enum: opMode  Value=opMode.DecrementHold  SampleTime=inf
  ec5 : simulink/Sources/Enumerated Constant  RequirementInfo={} %GIDa_0e7b19dd_d3b3_4e2c_bd65_1ecb5e9611f6  OutDataTypeStr=Enum: opMode  Value=opMode.Decrement  SampleTime=inf
  ec6 : simulink/Sources/Enumerated Constant  RequirementInfo={} %GIDa_f35bb6b6_3bef_45ef_99dd_5f19dbb4a7ec  OutDataTypeStr=Enum: reqMode  Value=reqMode.Cancel  SampleTime=inf
  ec7 : simulink/Sources/Enumerated Constant  RequirementInfo={} %GIDa_51a92104_4154_4f88_a119_bfbe5577d76f  OutDataTypeStr=Enum: opMode  Value=opMode.Resume  SampleTime=inf
  relop1 : RelationalOperator  RequirementInfo={} %GIDa_e29dc1b8_05cf_4e4c_8862_bdcd661f17f7  Operator===  OutDataTypeStr=boolean  InputSameDT=off
  relop2 : RelationalOperator  RequirementInfo={} %GIDa_1cfed6e8_7a4b_4da9_a8b9_d2aa9792081d  Operator===  OutDataTypeStr=boolean  InputSameDT=off
  relop3 : RelationalOperator  RequirementInfo={} %GIDa_6e684588_33a4_43bd_a988_859f8035445e  Operator===  OutDataTypeStr=boolean  InputSameDT=off
  relop4 : RelationalOperator  RequirementInfo={} %GIDa_dbbec9d9_1072_4193_8b48_0013e2a0af4a  Operator===  OutDataTypeStr=boolean  InputSameDT=off
  relop5 : RelationalOperator  RequirementInfo={} %GIDa_dfda4cb8_841e_4092_bf8e_9b454d549a3e  Operator===  OutDataTypeStr=boolean  InputSameDT=off
  relop6 : RelationalOperator  RequirementInfo={} %GIDa_7de70859_9d7b_4643_a601_1dc1b1cab207  Operator===  OutDataTypeStr=boolean  InputSameDT=off
  relop7 : RelationalOperator  RequirementInfo={} %GIDa_0d8b94db_b3c8_44c6_a54c_e24867b01db6  Operator===  OutDataTypeStr=boolean  InputSameDT=off
  yesno : Outport  RequirementInfo={} %GIDa_33cb442d_156f_49a0_ab01_e8b768f72bff  VectorParamsAs1DForOutWhenUnconnected=off
  wires:
  relop6/1 -> LogicOp2/6
  ec7/1 -> relop6/1
  relop7/1 -> LogicOp5/1
  LogicOp2/1 -> LogicOp5/2
  mode_prev/1 -> relop2/2, relop4/2, relop6/2, relop5/2, relop1/2, relop3/2
  reqDrv/1 -> relop7/2
  LogicOp5/1 -> yesno/1
  ec3/1 -> relop2/1
  ec2/1 -> relop3/1
  ec4/1 -> relop4/1
  ec5/1 -> relop5/1
  ec1/1 -> relop1/1
  relop5/1 -> LogicOp2/4
  relop4/1 -> LogicOp2/5
  relop3/1 -> LogicOp2/2
  relop2/1 -> LogicOp2/1
  relop1/1 -> LogicOp2/3
  ec6/1 -> relop7/1

== system CruiseControlMode/opMode/enableCondition/pressSetSw ==
  reqDrv : Inport  RequirementInfo={} %GIDa_0ae14d06_1ff5_46da_9a90_5f6ac958821d
  ec8 : simulink/Sources/Enumerated Constant  RequirementInfo={} %GIDa_f8d10115_ff1f_4e41_8891_2f92f5315ba5  OutDataTypeStr=Enum: reqMode  Value=reqMode.Cruise  SampleTime=inf
  relop6 : RelationalOperator  RequirementInfo={} %GIDa_6ead271e_2bff_463b_965f_7390f3e231c4  Operator===  OutDataTypeStr=boolean  InputSameDT=off
  yesno : Outport  RequirementInfo={} %GIDa_c7ccd60b_6e02_435a_8003_199c9914068a  VectorParamsAs1DForOutWhenUnconnected=off
  wires:
  relop6/1 -> yesno/1
  reqDrv/1 -> relop6/2
  ec8/1 -> relop6/1

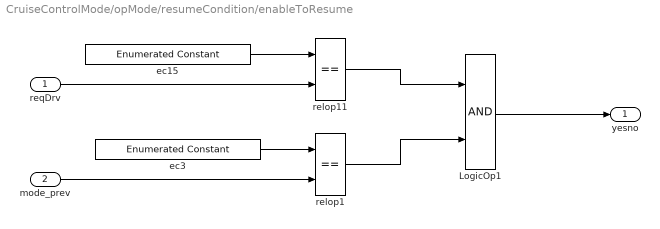
== system CruiseControlMode/opMode/resumeCondition/enableToResume ==
  reqDrv : Inport  RequirementInfo={} %GIDa_33009338_1281_41cb_8df0_1952db58348a
  mode_prev : Inport  RequirementInfo={} %GIDa_18fd4360_78fe_4c4c_afb7_0e5d14d120d5  Port=2
  LogicOp1 : Logic  RequirementInfo={} %GIDa_dd734ab8_97ca_4e92_9889_b70d3d29659b  AllPortsSameDT=off  OutDataTypeStr=boolean
  ec15 : simulink/Sources/Enumerated Constant  RequirementInfo={} %GIDa_9a0373aa_46b5_43e3_9c45_6b251c1b8ba6  OutDataTypeStr=Enum: reqMode  Value=reqMode.ResumeReq  SampleTime=inf
  ec3 : simulink/Sources/Enumerated Constant  RequirementInfo={} %GIDa_024b2391_093d_4079_95c0_a4c5171015b4  OutDataTypeStr=Enum: opMode  Value=opMode.Enable  SampleTime=inf
  relop1 : RelationalOperator  RequirementInfo={} %GIDa_98adee4d_e89f_4413_a8ec_6982af447914  Operator===  OutDataTypeStr=boolean  InputSameDT=off
  relop11 : RelationalOperator  RequirementInfo={} %GIDa_490cc3d2_b969_4361_a465_8476d3daa15b  Operator===  OutDataTypeStr=boolean  InputSameDT=off
  yesno : Outport  RequirementInfo={} %GIDa_3d078793_2fd4_4e28_8f7c_2c07ef2360b8  VectorParamsAs1DForOutWhenUnconnected=off
  wires:
  LogicOp1/1 -> yesno/1
  ec3/1 -> relop1/1
  relop1/1 -> LogicOp1/2
  mode_prev/1 -> relop1/2
  relop11/1 -> LogicOp1/1
  reqDrv/1 -> relop11/2
  ec15/1 -> relop11/1

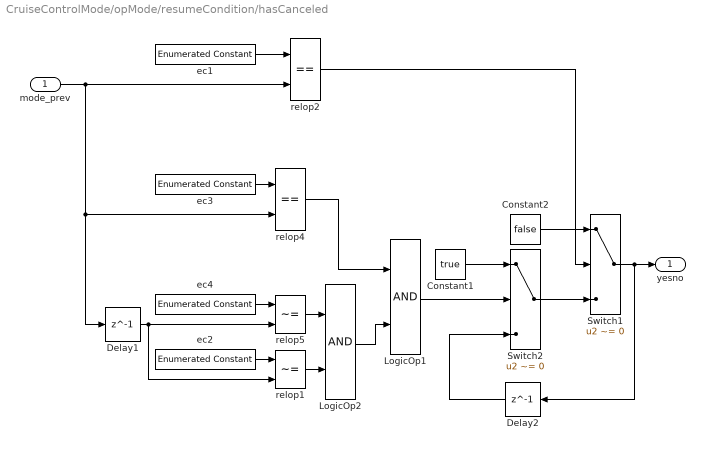
== system CruiseControlMode/opMode/resumeCondition/hasCanceled ==
  mode_prev : Inport  RequirementInfo={} %GIDa_c239aeb4_7db9_4fd5_abca_888541b23c4b
  Constant1 : Constant  RequirementInfo={} %GIDa_51c6ff93_ed4c_446a_bfcf_4a84e4bb89f5  Value=true  OutDataTypeStr=boolean
  Constant2 : Constant  RequirementInfo={} %GIDa_4350d5f5_a654_4520_8531_5d5d27b56ad5  Value=false  OutDataTypeStr=boolean
  Delay1 : Delay  RequirementInfo={} %GIDa_69d36855_dfc2_4ecb_9c86_9a0d2fba9a9b  DelayLength=1  InitialCondition=opMode.Disable
      settings: AttributesFormatString=Init=%<InitialCondition>
  Delay2 : Delay  RequirementInfo={} %GIDa_a1165942_49b8_4efa_aee6_936ba84eab2b  DelayLength=1  InitialCondition=false
      settings: AttributesFormatString=Init=%<InitialCondition>
  LogicOp1 : Logic  RequirementInfo={} %GIDa_efb24f8b_9975_42ee_869c_3a918466a712  AllPortsSameDT=off  OutDataTypeStr=boolean
  LogicOp2 : Logic  RequirementInfo={} %GIDa_aa3c69de_1f21_404c_9ca9_6e8f1b230840  AllPortsSameDT=off  OutDataTypeStr=boolean
  Switch1 : Switch  RequirementInfo={} %GIDa_90908c4b_5fa4_46b2_97c2_bc966ffbb382  Criteria=u2 ~= 0  SaturateOnIntegerOverflow=off  InputSameDT=off
  Switch2 : Switch  RequirementInfo={} %GIDa_955cbbb7_6948_4c6c_9b81_a647a5cbc21c  Criteria=u2 ~= 0  SaturateOnIntegerOverflow=off  InputSameDT=off
  ec1 : simulink/Sources/Enumerated Constant  RequirementInfo={} %GIDa_c1442db7_1d8b_427d_a163_c7046a2cac4e  OutDataTypeStr=Enum: opMode  Value=opMode.Disable  SampleTime=inf
  ec2 : simulink/Sources/Enumerated Constant  RequirementInfo={} %GIDa_aa487a31_a88e_4007_a8ff_d50aea5db727  OutDataTypeStr=Enum: opMode  Value=opMode.Enable  SampleTime=inf
  ec3 : simulink/Sources/Enumerated Constant  RequirementInfo={} %GIDa_c2911e92_c1e0_434b_8250_ad0e97354cfc  OutDataTypeStr=Enum: opMode  Value=opMode.Enable  SampleTime=inf
  ec4 : simulink/Sources/Enumerated Constant  RequirementInfo={} %GIDa_429cdb1c_8adf_406e_b187_0ab9a24d78be  OutDataTypeStr=Enum: opMode  Value=opMode.Disable  SampleTime=inf
  relop1 : RelationalOperator  RequirementInfo={} %GIDa_e0f3aa3f_7828_4b3b_ae42_9788052a5c27  Operator=~=  OutDataTypeStr=boolean  InputSameDT=off
  relop2 : RelationalOperator  RequirementInfo={} %GIDa_4b5feb9d_1c2e_4310_ba70_d7162ff450e0  Operator===  OutDataTypeStr=boolean  InputSameDT=off
  relop4 : RelationalOperator  RequirementInfo={} %GIDa_a99a828c_935a_4baf_9b3d_02095dbe4275  Operator===  OutDataTypeStr=boolean  InputSameDT=off
  relop5 : RelationalOperator  RequirementInfo={} %GIDa_aec82208_3e8f_461d_b387_6a00b96d6eee  Operator=~=  OutDataTypeStr=boolean  InputSameDT=off
  yesno : Outport  RequirementInfo={} %GIDa_242d0d0a_da28_4fb9_af46_c99ad7214268  VectorParamsAs1DForOutWhenUnconnected=off
  wires:
  Delay1/1 -> relop5/2, relop1/2
  LogicOp2/1 -> LogicOp1/2
  relop1/1 -> LogicOp2/2
  relop5/1 -> LogicOp2/1
  ec2/1 -> relop1/1
  mode_prev/1 -> relop4/2, Delay1/1, relop2/2
  ec1/1 -> relop2/1
  relop2/1 -> Switch1/2
  Switch2/1 -> Switch1/3
  Constant2/1 -> Switch1/1
  Switch1/1 -> Delay2/1, yesno/1
  relop4/1 -> LogicOp1/1
  Constant1/1 -> Switch2/1
  Delay2/1 -> Switch2/3
  LogicOp1/1 -> Switch2/2
  ec4/1 -> relop5/1
  ec3/1 -> relop4/1

== system CruiseControlMode/opMode/activateCondition/waitingForButtonHolding/ec10 ==
  Constant : Constant  RequirementInfo={} %GIDa_5970f669_49a7_4e77_ab6d_b745af3717b8  DialogController=Simulink.DDGSource  Value=reqMode.Dec_Middle  OutDataTypeStr=Enum: reqMode  LockScale=on
  Out : Outport  RequirementInfo={} %GIDa_1b5b0287_3214_4608_a9bb_77440b889f0f  VectorParamsAs1DForOutWhenUnconnected=off
  wires:
  Constant/1 -> Out/1

== system CruiseControlMode/opMode/activateCondition/waitingForButtonHolding/ec8 ==
  Constant : Constant  RequirementInfo={} %GIDa_e66d3b00_4861_4957_ac0a_d253c75ee4c1  DialogController=Simulink.DDGSource  Value=reqMode.Inc_Middle  OutDataTypeStr=Enum: reqMode  LockScale=on
  Out : Outport  RequirementInfo={} %GIDa_eb65c83d_b8e7_4d0d_9021_c8611bf7d074  VectorParamsAs1DForOutWhenUnconnected=off
  wires:
  Constant/1 -> Out/1
